simulink model "P6simulink"  (R2025a)
settings: Solver=ode23  StartTime=0.0  StopTime=0.01  RelTol=1e-3
model workspace (MAT data in the model file):
  C = 1e-05
  L = 0.002
  R = 10
  Uin = 32
settings Model: Creator=DELL  LastModifiedBy=ernes

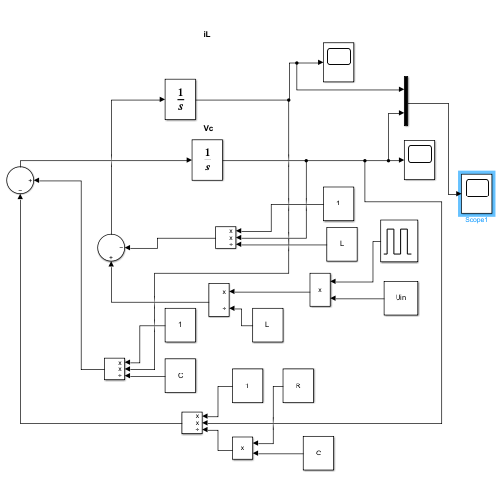
[thumbnail: Simulink's stored preview of the top-level diagram]
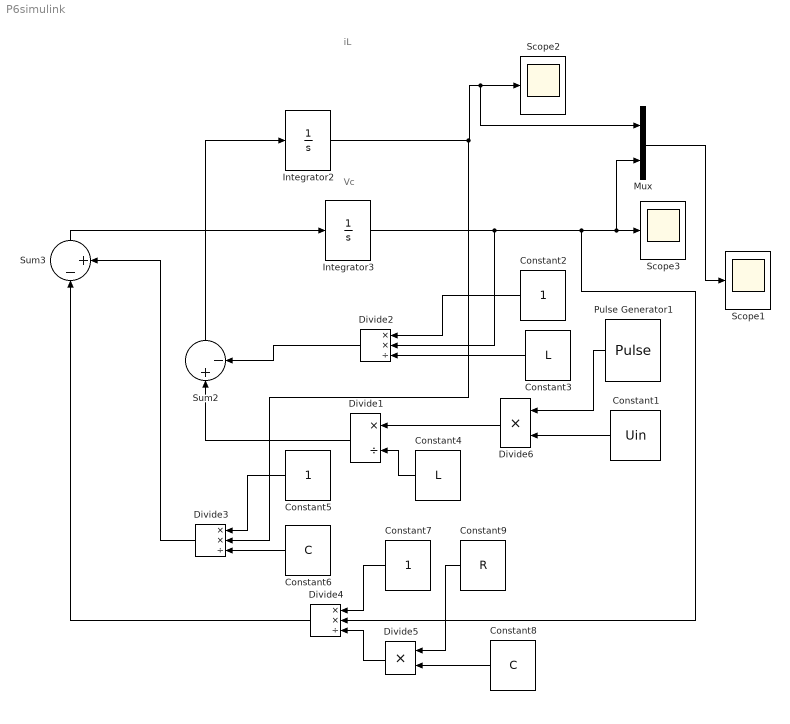
== system P6simulink ==
  note: Vc
  note: iL
  Constant1 : Constant  Value=Uin
  Constant2 : Constant
  Constant3 : Constant  Value=L
  Constant4 : Constant  Value=L
  Constant5 : Constant
  Constant6 : Constant  Value=C
  Constant7 : Constant
  Constant8 : Constant  Value=C
  Constant9 : Constant  Value=R
  Divide1 : Product  Inputs=*/
  Divide2 : Product  Inputs=**/
  Divide3 : Product  Inputs=**/
  Divide4 : Product  Inputs=**/
  Divide5 : Product  Inputs=**
  Divide6 : Product  Inputs=**
  Integrator2 : Integrator
  Integrator3 : Integrator
  Mux : Mux  Inputs=2
  Pulse Generator1 : DiscretePulseGenerator  PulseType=Time based  Period=1e-5  PulseWidth=40
  Scope1 : Scope
      settings: ActiveDisplayYMinimum=-0.12455196763692078  ActiveDisplayYMaximum=1.5242194609345074
  Scope2 : Scope
      settings: ActiveDisplayYMinimum=-0.17312  ActiveDisplayYMaximum=1.55809
  Scope3 : Scope
      settings: ActiveDisplayYMinimum=3.36858  ActiveDisplayYMaximum=14.49578  DataLoggingVariableName=ScopeData2
  Sum2 : Sum  Inputs=|+-
  Sum3 : Sum  Inputs=|-+
  wires:
  Integrator2/1 -> Mux/1, Scope2/1, Divide3/2
  Sum3/1 -> Integrator3/1
  Sum2/1 -> Integrator2/1
  Constant3/1 -> Divide2/3
  Constant2/1 -> Divide2/1
  Integrator3/1 -> Divide4/2, Mux/2, Scope3/1, Divide2/2
  Divide2/1 -> Sum2/2
  Divide1/1 -> Sum2/1
  Constant5/1 -> Divide3/1
  Constant6/1 -> Divide3/3
  Divide3/1 -> Sum3/2
  Constant7/1 -> Divide4/1
  Constant9/1 -> Divide5/1
  Constant8/1 -> Divide5/2
  Divide5/1 -> Divide4/3
  Divide4/1 -> Sum3/1
  Pulse Generator1/1 -> Divide6/1
  Divide6/1 -> Divide1/1
  Constant4/1 -> Divide1/2
  Constant1/1 -> Divide6/2
  Mux/1 -> Scope1/1
